simulink library "MCHP_Blockset"  (R2014b)
settings: Solver=ode45  SolverMode=SingleTasking  StartTime=0.0  StopTime=10.0  RelTol=1e-3
InitFcn:
  | disp('MCHP_Blockset_Library_InitFunction');
undefined symbols (not defined in the file): A0, A2, AD0, AVdd, B1, B5, B9, C10, C2, CMP2A, CMP3A, CMP4A, EXTREF1, EXTREF2, gcbh, MaxPer, MCHP_ACC_SAMx_Callback, MCHP_ADC_Callback, MCHP_ADC_HighSpeed_SAR_Callback, MCHP_ADC_HighSpeed_SAR_dsPIC_Callback, MCHP_ADC_SAME5x_Callback, MCHP_AFEC_SAM7x_Callback, MCHP_BUS_I2C_MASTER_callback, MCHP_BUS_SPI_callback, MCHP_C_function_Call_callback, MCHP_CN_Callback, MCHP_COMPARATOR1_callback, MCHP_CompilerOptimisation_Callback, MCHP_DACC_SAMx_Callback, MCHP_Digital_Input_Callback, MCHP_Digital_Output_Read_Callback, MCHP_Digital_Output_Write_Callback, MCHP_Fun, MCHP_HighSpeed_AnalogComparator_Callback, MCHP_IC_Callback, MCHP_IdleTask_Callback, MCHP_Interrupt_Callback, MCHP_Master_Callback, MCHP_MCPWM_Callback, MCHP_MCU_LOAD_Callback, MCHP_MCU_OVERLOAD_Callback, MCHP_MSI_Callback, MCHP_OC_HW_Callback, MCHP_OC_SW_Callback, MCHP_OP_AMP_Callback, MCHP_OrderInOut, MCHP_PDEC_Callback, MCHP_PGA_Callback, MCHP_PWM_Callback, MCHP_PWM_HighSpeed_Override_Callback, MCHP_PWM_HS_FEP_Callback, MCHP_PWM_SAM7x_Callback, MCHP_PWM_SAM7x_Override_Callback, MCHP_QDEC_SAMx_Callback, MCHP_QEI_Callback, MCHP_Scheduler_Options_Callback, MCHP_SECONDARY_CORE_Callback, MCHP_Tasks_State_Callback, MCHP_TCC_PWM_Callback, MCHP_TIMER_Config_Callback ... (+18)
libraries: MCHP_Blockset x2
(part 7 of 9)

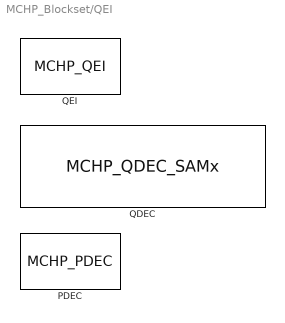
== system MCHP_Blockset/QEI ==
  PDEC : S-Function  InitFcn=MCHP_PDEC_Callback(gcb,'InitFcn');  FunctionName=MCHP_PDEC  Parameters=MCHP_PDEC_Callback(gcbh,'S_INPUT'),MCHP_PDEC_Callback(gcbh,'S_OUTPUT'),MCHP_PDEC_Callback(gcbh,'S_INPUT_Size'),MCHP_PDEC_Callback(gcbh,'S_OUTPUT_Size'),MCHP_PDEC_Callback(gcbh,'S_ListCustomDatatype'),SampleTime,0  EnableBusSupport=off  mask(PDEC){Mode=Quadrature Encoder, index=Reset counter, QDI0=PC16 / Pin[70], QDI0_txt=Dynamic Options, QDI1=PC17 / Pin[71], QDI1_txt=Dynamic Options, QDI2=PC18 / Pin[72], QDI2_txt=Dynamic Options, maxCounterReset=500, AutoCorrection=on, AutoCorrection_override=on, info=0, MCHP_MASTERLINK=SAME5x_PDEC_QEI_R2014b/Microchip Master, SampleTime=.01, MCHP_PORT={PDEC A}{QDI0}5:0:P80;{PDEC B}{QDI1}5:0:P81;{PDEC index}{QDI2}5:0:P82;, MAXPOS_INPUT=off, RESET_INPUT=off, OutputCounter=on, OutputCounter_Signed=unsigned, OutputRevolution=off, CounterRevolution_length=Counter is 13 bits ; revolution is 3 bits, OutputRevolution_Signed=unsigned, FILTER=2.55 (us)  ->  freq 196 (KHz), FILTER_TXT=2.55 (us)  ->  freq 196 (KHz), SWAP=off, QDI_invert_0=off, QDI_invert_1=off, QDI_invert_2=off}
      mask prompts: QDI0 "Phase A (QDI0)"; QDI0_txt "Signal 0"; QDI1 "Phase B (QDO1)"; QDI1_txt "Signal 1"; QDI2 "Index (QDI2)"; QDI2_txt "Signal 2"; maxCounterReset "Reset counter at value (-1 for never)"; AutoCorrection "Enable Auto-correction"; AutoCorrection_override "Enable Auto-correction"; SampleTime "Sample Time"; MAXPOS_INPUT "Max Counter is a block input"; RESET_INPUT "Reset Position and Counter on block input level"; OutputCounter "Output counter value"; OutputCounter_Signed "Output counter is"; OutputRevolution "Output revolution"; CounterRevolution_length "Length"; OutputRevolution_Signed "Output revolution is"; FILTER "Filter: min signal duration"; FILTER_TXT "Filter inputs"; SWAP "Swap pin phase A && B"; QDI_invert_0 "Invert Phase A logic (QDI0)"; QDI_invert_1 "Invert Phase B logic (QDI1)"; QDI_invert_2 "Invert index logic (QDI2)"
      mask help:
      | PDEC peripheral for SAM D5x / E5x / PIC32C
      |
      | Quadrature Encoder
      mask init:
      | MCHP_PDEC_Callback(gcbh,'INITIALISATION');
      settings: CopyFcn=MCHP_Fun.BlockUpdate(gcbh);  DeleteFcn=MCHP_PDEC_Callback(gcbh,'DeleteFcn');  OpenFcn=MCHP_PDEC_Callback(gcb,'OPEN');
      mask TypeOptions Mode: Quadrature Encoder | Counter with direction
      mask Callback Mode: MCHP_PDEC_Callback(gcbh,'UpdateGUI');
      mask TypeOptions index: Not used | Reset counter
      mask Callback index: MCHP_PDEC_Callback(gcbh,'UpdateGUI');
      mask TypeOptions QDI0: PA24 / Pin[94] | PB18 / Pin[84] | PB23 / Pin[99] | PC16 / Pin[70]
      mask TypeOptions QDI0_txt: Dynamic Options
      mask TypeOptions QDI1: PA25 / Pin[95] | PB19 / Pin[85] | PB24 / Pin[100] | PC17 / Pin[71]
      mask TypeOptions QDI1_txt: Dynamic Options
      mask TypeOptions QDI2: PB20 / Pin[86] | PB22 / Pin[98] | PB25 / Pin[101] | PC18 / Pin[72]
      mask TypeOptions QDI2_txt: Dynamic Options
      mask Callback MAXPOS_INPUT: MCHP_PDEC_Callback(gcbh,'UpdateGUI');
      mask TypeOptions OutputCounter_Signed: unsigned | signed
      mask Callback OutputRevolution: MCHP_PDEC_Callback(gcbh,'UpdateGUI');
      mask TypeOptions CounterRevolution_length: Counter is 16 bits ; no revolution | Counter is 15 bits ; revolution is 1 bit | Counter is 14 bits ; revolution is 2 bits | Counter is 13 bits ; revolution is 3 bits | Counter is 12 bits ; revolution is 4 bits | Counter is 11 bits ; revolution is 5 bits | Counter is 10 bits ; revolution is 6 bits | Counter is   9 bits ; revolution is 7 bits
      mask Callback CounterRevolution_length: MCHP_PDEC_Callback(gcbh,'UpdateGUI');
      mask TypeOptions OutputRevolution_Signed: unsigned | signed
      mask TypeOptions FILTER: disabled | 10 (ns)  ->  freq 50 (MHz) | 20 (ns)  ->  freq 25 (MHz) | 30 (ns)  ->  freq 16.7 (MHz) | 40 (ns)  ->  freq 12.5 (MHz) | 50 (ns)  ->  freq 10 (MHz) | 60 (ns)  ->  freq 8.33 (MHz) | 70 (ns)  ->  freq 7.14 (MHz) | 80 (ns)  ->  freq 6.25 (MHz) | 90 (ns)  ->  freq 5.56 (MHz) | 100 (ns)  ->  freq 5 (MHz) | 110 (ns)  ->  freq 4.55 (MHz) | 120 (ns)  ->  freq 4.17 (MHz) | 130 (ns)  ->  freq 3.85 (MHz) | 140 (ns)  ->  freq 3.57 (MHz) | 150 (ns)  ->  freq 3.33 (MHz) | 160 (ns)  ->  freq 3.13 (MHz) | 170 (ns)  ->  freq 2.94 (MHz) | 180 (ns)  ->  freq 2.78 (MHz) | 190 (ns)  ->  freq 2.63 (MHz) | 200 (ns)  ->  freq 2.5 (MHz) | 210 (ns)  ->  freq 2.38 (MHz) | 220 (ns)  ->  freq 2.27 (MHz) | 230 (ns)  ->  freq 2.17 (MHz) | 240 (ns)  ->  freq 2.08 (MHz) | 250 (ns)  ->  freq 2 (MHz) | 260 (ns)  ->  freq 1.92 (MHz) | 270 (ns)  ->  freq 1.85 (MHz) | 280 (ns)  ->  freq 1.79 (MHz) | 290 (ns)  ->  freq 1.72 (MHz) | 300 (ns)  ->  freq 1.67 (MHz) | 310 (ns)  ->  freq 1.61 (MHz) | 320 (ns)  ->  freq 1.56 (MHz) | 330 (ns)  ->  freq 1.52 (MHz) | 340 (ns)  ->  freq 1.47 (MHz) | 350 (ns)  ->  freq 1.43 (MHz) | 360 (ns)  ->  freq 1.39 (MHz) | 370 (ns)  ->  freq 1.35 (MHz) | 380 (ns)  ->  freq 1.32 (MHz) | 390 (ns)  ->  freq 1.28 (MHz) | 400 (ns)  ->  freq 1.25 (MHz) | 410 (ns)  ->  freq 1.22 (MHz) | 420 (ns)  ->  freq 1.19 (MHz) | 430 (ns)  ->  freq 1.16 (MHz) | 440 (ns)  ->  freq 1.14 (MHz) | 450 (ns)  ->  freq 1.11 (MHz) | 460 (ns)  ->  freq 1.09 (MHz) | 470 (ns)  ->  freq 1.06 (MHz) | 480 (ns)  ->  freq 1.04 (MHz) | 490 (ns)  ->  freq 1.02 (MHz) | 500 (ns)  ->  freq 1e+03 (KHz) | 510 (ns)  ->  freq 980 (KHz) | 520 (ns)  ->  freq 962 (KHz) | 530 (ns)  ->  freq 943 (KHz) | 540 (ns)  ->  freq 926 (KHz) | 550 (ns)  ->  freq 909 (KHz) | 560 (ns)  ->  freq 893 (KHz) | 570 (ns)  ->  freq 877 (KHz) | 580 (ns)  ->  freq 862 (KHz) | 590 (ns)  ->  freq 847 (KHz) | 600 (ns)  ->  freq 833 (KHz) | 610 (ns)  ->  freq 820 (KHz) | 620 (ns)  ->  freq 806 (KHz) | 630 (ns)  ->  freq 794 (KHz) | 640 (ns)  ->  freq 781 (KHz) | 650 (ns)  ->  freq 769 (KHz) | 660 (ns)  ->  freq 758 (KHz) | 670 (ns)  ->  freq 746 (KHz) | 680 (ns)  ->  freq 735 (KHz) | 690 (ns)  ->  freq 725 (KHz) | 700 (ns)  ->  freq 714 (KHz) | 710 (ns)  ->  freq 704 (KHz) | 720 (ns)  ->  freq 694 (KHz) | 730 (ns)  ->  freq 685 (KHz) | 740 (ns)  ->  freq 676 (KHz) | 750 (ns)  ->  freq 667 (KHz) | 760 (ns)  ->  freq 658 (KHz) | 770 (ns)  ->  freq 649 (KHz) | 780 (ns)  ->  freq 641 (KHz) | 790 (ns)  ->  freq 633 (KHz) | 800 (ns)  ->  freq 625 (KHz) | 810 (ns)  ->  freq 617 (KHz) | 820 (ns)  ->  freq 610 (KHz) | 830 (ns)  ->  freq 602 (KHz) | 840 (ns)  ->  freq 595 (KHz) | 850 (ns)  ->  freq 588 (KHz) | 860 (ns)  ->  freq 581 (KHz) | 870 (ns)  ->  freq 575 (KHz) | 880 (ns)  ->  freq 568 (KHz) | 890 (ns)  ->  freq 562 (KHz) | 900 (ns)  ->  freq 556 (KHz) | 910 (ns)  ->  freq 549 (KHz) | 920 (ns)  ->  freq 543 (KHz) | 930 (ns)  ->  freq 538 (KHz) | 940 (ns)  ->  freq 532 (KHz) | 950 (ns)  ->  freq 526 (KHz) | 960 (ns)  ->  freq 521 (KHz) | 970 (ns)  ->  freq 515 (KHz) | 980 (ns)  ->  freq 510 (KHz) | 990 (ns)  ->  freq 505 (KHz) | 1e+03 (ns)  ->  freq 500 (KHz) | 1.01 (us)  ->  freq 495 (KHz) | 1.02 (us)  ->  freq 490 (KHz) | 1.03 (us)  ->  freq 485 (KHz) | 1.04 (us)  ->  freq 481 (KHz) | 1.05 (us)  ->  freq 476 (KHz) | 1.06 (us)  ->  freq 472 (KHz) | 1.07 (us)  ->  freq 467 (KHz) | 1.08 (us)  ->  freq 463 (KHz) | 1.09 (us)  ->  freq 459 (KHz) | 1.1 (us)  ->  freq 455 (KHz) | 1.11 (us)  ->  freq 450 (KHz) | 1.12 (us)  ->  freq 446 (KHz) | 1.13 (us)  ->  freq 442 (KHz) | 1.14 (us)  ->  freq 439 (KHz) | 1.15 (us)  ->  freq 435 (KHz) | 1.16 (us)  ->  freq 431 (KHz) | 1.17 (us)  ->  freq 427 (KHz) | 1.18 (us)  ->  freq 424 (KHz) | 1.19 (us)  ->  freq 420 (KHz) | 1.2 (us)  ->  freq 417 (KHz) | 1.21 (us)  ->  freq 413 (KHz) | 1.22 (us)  ->  freq 410 (KHz) | 1.23 (us)  ->  freq 407 (KHz) | 1.24 (us)  ->  freq 403 (KHz) | 1.25 (us)  ->  freq 400 (KHz) | 1.26 (us)  ->  freq 397 (KHz) | 1.27 (us)  ->  freq 394 (KHz) | 1.28 (us)  ->  freq 391 (KHz) | 1.29 (us)  ->  freq 388 (KHz) | 1.3 (us)  ->  freq 385 (KHz) | 1.31 (us)  ->  freq 382 (KHz) | 1.32 (us)  ->  freq 379 (KHz) | 1.33 (us)  ->  freq 376 (KHz) | 1.34 (us)  ->  freq 373 (KHz) | 1.35 (us)  ->  freq 370 (KHz) | 1.36 (us)  ->  freq 368 (KHz) | 1.37 (us)  ->  freq 365 (KHz) | 1.38 (us)  ->  freq 362 (KHz) | 1.39 (us)  ->  freq 360 (KHz) | 1.4 (us)  ->  freq 357 (KHz) | 1.41 (us)  ->  freq 355 (KHz) | 1.42 (us)  ->  freq 352 (KHz) | 1.43 (us)  ->  freq 350 (KHz) | 1.44 (us)  ->  freq 347 (KHz) | 1.45 (us)  ->  freq 345 (KHz) | 1.46 (us)  ->  freq 342 (KHz) | 1.47 (us)  ->  freq 340 (KHz) | 1.48 (us)  ->  freq 338 (KHz) | 1.49 (us)  ->  freq 336 (KHz) | 1.5 (us)  ->  freq 333 (KHz) | 1.51 (us)  ->  freq 331 (KHz) | 1.52 (us)  ->  freq 329 (KHz) | 1.53 (us)  ->  freq 327 (KHz) | 1.54 (us)  ->  freq 325 (KHz) | 1.55 (us)  ->  freq 323 (KHz) | 1.56 (us)  ->  freq 321 (KHz) | 1.57 (us)  ->  freq 318 (KHz) | 1.58 (us)  ->  freq 316 (KHz) | 1.59 (us)  ->  freq 314 (KHz) | 1.6 (us)  ->  freq 313 (KHz) | 1.61 (us)  ->  freq 311 (KHz) | 1.62 (us)  ->  freq 309 (KHz) | 1.63 (us)  ->  freq 307 (KHz) | 1.64 (us)  ->  freq 305 (KHz) | 1.65 (us)  ->  freq 303 (KHz) | 1.66 (us)  ->  freq 301 (KHz) | 1.67 (us)  ->  freq 299 (KHz) | 1.68 (us)  ->  freq 298 (KHz) | 1.69 (us)  ->  freq 296 (KHz) | 1.7 (us)  ->  freq 294 (KHz) | 1.71 (us)  ->  freq 292 (KHz) | 1.72 (us)  ->  freq 291 (KHz) | 1.73 (us)  ->  freq 289 (KHz) | 1.74 (us)  ->  freq 287 (KHz) | 1.75 (us)  ->  freq 286 (KHz) | 1.76 (us)  ->  freq 284 (KHz) | 1.77 (us)  ->  freq 282 (KHz) | 1.78 (us)  ->  freq 281 (KHz) | 1.79 (us)  ->  freq 279 (KHz) | 1.8 (us)  ->  freq 278 (KHz) | 1.81 (us)  ->  freq 276 (KHz) | 1.82 (us)  ->  freq 275 (KHz) | 1.83 (us)  ->  freq 273 (KHz) | 1.84 (us)  ->  freq 272 (KHz) | 1.85 (us)  ->  freq 270 (KHz) | 1.86 (us)  ->  freq 269 (KHz) | 1.87 (us)  ->  freq 267 (KHz) | 1.88 (us)  ->  freq 266 (KHz) | 1.89 (us)  ->  freq 265 (KHz) | 1.9 (us)  ->  freq 263 (KHz) | 1.91 (us)  ->  freq 262 (KHz) | 1.92 (us)  ->  freq 260 (KHz) | 1.93 (us)  ->  freq 259 (KHz) | 1.94 (us)  ->  freq 258 (KHz) | 1.95 (us)  ->  freq 256 (KHz) | 1.96 (us)  ->  freq 255 (KHz) | 1.97 (us)  ->  freq 254 (KHz) | 1.98 (us)  ->  freq 253 (KHz) | 1.99 (us)  ->  freq 251 (KHz) | 2 (us)  ->  freq 250 (KHz) | 2.01 (us)  ->  freq 249 (KHz) | 2.02 (us)  ->  freq 248 (KHz) | 2.03 (us)  ->  freq 246 (KHz) | 2.04 (us)  ->  freq 245 (KHz) | 2.05 (us)  ->  freq 244 (KHz) | 2.06 (us)  ->  freq 243 (KHz) | 2.07 (us)  ->  freq 242 (KHz) | 2.08 (us)  ->  freq 240 (KHz) | 2.09 (us)  ->  freq 239 (KHz) | 2.1 (us)  ->  freq 238 (KHz) | 2.11 (us)  ->  freq 237 (KHz) | 2.12 (us)  ->  freq 236 (KHz) | 2.13 (us)  ->  freq 235 (KHz) | 2.14 (us)  ->  freq 234 (KHz) | 2.15 (us)  ->  freq 233 (KHz) | 2.16 (us)  ->  freq 231 (KHz) | 2.17 (us)  ->  freq 230 (KHz) | 2.18 (us)  ->  freq 229 (KHz) | 2.19 (us)  ->  freq 228 (KHz) | 2.2 (us)  ->  freq 227 (KHz) | 2.21 (us)  ->  freq 226 (KHz) | 2.22 (us)  ->  freq 225 (KHz) | 2.23 (us)  ->  freq 224 (KHz) | 2.24 (us)  ->  freq 223 (KHz) | 2.25 (us)  ->  freq 222 (KHz) | 2.26 (us)  ->  freq 221 (KHz) | 2.27 (us)  ->  freq 220 (KHz) | 2.28 (us)  ->  freq 219 (KHz) | 2.29 (us)  ->  freq 218 (KHz) | 2.3 (us)  ->  freq 217 (KHz) | 2.31 (us)  ->  freq 216 (KHz) | 2.32 (us)  ->  freq 216 (KHz) | 2.33 (us)  ->  freq 215 (KHz) | 2.34 (us)  ->  freq 214 (KHz) | 2.35 (us)  ->  freq 213 (KHz) | 2.36 (us)  ->  freq 212 (KHz) | 2.37 (us)  ->  freq 211 (KHz) | 2.38 (us)  ->  freq 210 (KHz) | 2.39 (us)  ->  freq 209 (KHz) | 2.4 (us)  ->  freq 208 (KHz) | 2.41 (us)  ->  freq 207 (KHz) | 2.42 (us)  ->  freq 207 (KHz) | 2.43 (us)  ->  freq 206 (KHz) | 2.44 (us)  ->  freq 205 (KHz) | 2.45 (us)  ->  freq 204 (KHz) | 2.46 (us)  ->  freq 203 (KHz) | 2.47 (us)  ->  freq 202 (KHz) | 2.48 (us)  ->  freq 202 (KHz) | 2.49 (us)  ->  freq 201 (KHz) | 2.5 (us)  ->  freq 200 (KHz) | 2.51 (us)  ->  freq 199 (KHz) | 2.52 (us)  ->  freq 198 (KHz) | 2.53 (us)  ->  freq 198 (KHz) | 2.54 (us)  ->  freq 197 (KHz) | 2.55 (us)  ->  freq 196 (KHz)
      mask Display:
      | MCHP_DrawLogo;fprintf('PDEC');
      | port_label('output', 1 ,' count ');
  QDEC : S-Function  InitFcn=MCHP_QDEC_SAMx_Callback(gcbh,'InitFcn');  FunctionName=MCHP_QDEC_SAMx  Parameters=MCHP_QDEC_SAMx_Callback(gcbh,'S_INPUT'),MCHP_QDEC_SAMx_Callback(gcbh,'S_OUTPUT'),MCHP_QDEC_SAMx_Callback(gcbh,'S_INPUT_Size'),MCHP_QDEC_SAMx_Callback(gcbh,'S_OUTPUT_Size'),MCHP_QDEC_SAMx_Callback(gcbh,'S_INPUT_FeedThrough'),0,SampleTime,0  EnableBusSupport=off  mask(Ouput Driver for Quadrature Decoder (QDEC)){QDEC_REF=Dynamic Options, QDEC_REF_TXT=TC0, PHA_PIN=Dynamic Options, PHA_PIN_TXT=PA0 / Pin[102], PHB_PIN=Dynamic Options, PHB_PIN_TXT=PA1 / Pin[99], IDX_PIN=Dynamic Options, IDX_PIN_TXT=PA16 / Pin[45], INVERT_PHA=off, INVERT_PHB=off, INVERT_IDX=on, SWAP_PHA_PHB=off, SampleTime=.001, MCHP_PORT={TC0}{TIOA0}3:0:P0;{TC0}{TIOB0}3:0:P1;{TC0}{TIOB1}3:0:P16;, MCHP_MASTERLINK=SAMx7_MCLV2_QDEC_Testing_R2014b/Microchip Master, MCHP_TIMER_REQUEST={Quadrature Decoder (Phase Counter)}{QDEC0}20:4:4:0:[1]:65535;{Quadrature Decoder (IDX Counter)}{QDEC0}20:4:4:0:[2]:65535;{Quadrature Decoder (Speed Measurement Time Base)}{QDEC0}20:4:4:0:[3]:65535;, MCHP_TIMER_RESULT=[0 -0.5 ;2 65533.999999999985448 ;3 65533.999999999985448 ], QDEC_MODE=Position, POSITION_OUTPUT=is a 16 bits signed block output, INDEX_OUTPUT=is not a block output, RESET_INPUT=off, POSITION_RESET_MODE=on each IDX signal, RESET_EDGE=rising edge, POSITION_RESET_VALUE=1000, SPEED_TIME_BASE=Dynamic Options, SPEED_TIME_BASE_TXT=Resol: 666.7(ns) - MaxPer: 43.7(ms), SPEED_OUTPUT=is a 16 bits unsigned block output, DIR_OUTPUT=is a boolean block output, DIRCHG_OUTPUT=is a boolean block output, AUTO_CORRECTION=on, MAX_PERIOD_FILTER=Dynamic Options, MAX_PERIOD_FILTER_TXT=4(us), MAXCMP=disabled, MPE_OUTPUT=is not a block output, QERR_OUTPUT=is not a block output}
      mask prompts: QDEC_REF "QDEC set on Timer Counter"; QDEC_REF_TXT "QDEC_REF"; PHA_PIN "Phase A Input Signal (PHA)"; PHB_PIN "Phase B Input Signal (PHB)"; IDX_PIN "Index Input Signal (IDX)"; INVERT_PHA "Invert PHA"; INVERT_PHB "Invert PHB"; INVERT_IDX "Invert IDX"; SWAP_PHA_PHB "Swap PHA and PHB"; SampleTime "Sample Time"; QDEC_MODE "QDEC Mode"; POSITION_OUTPUT "Pulse Counter (Absolute Position)"; INDEX_OUTPUT "Index Counter (Number of rotations)"; RESET_INPUT "Reset Position and Index Counters on block input level"; POSITION_RESET_MODE "Position Reset Mode"; RESET_EDGE "Reset Position on IDX signal"; POSITION_RESET_VALUE "Position Reset Value  (range [0  65535])"; SPEED_TIME_BASE "Speed Measurement time base"; SPEED_TIME_BASE_TXT "SPEED_TIME_BASE"; SPEED_OUTPUT "Speed"; DIR_OUTPUT "Direction Status"; DIRCHG_OUTPUT "Rotation Change Detection Flag"; AUTO_CORRECTION "Enable AutoCorrection of missing pulses"; MAX_PERIOD_FILTER "Filter phase pulses with a period shorter than"; MAXCMP "Maximum Consecutive Missing Pulses allowed"; MPE_OUTPUT "Consecutive Missing Pulse Error Flag"; QERR_OUTPUT "Quadrature Error Flag"
      mask help:
      | The Quadrature Decoder (QDEC) is connected in front of the Timer-Counter module (TC). When enabled, the QDEC performs the input lines filtering, decoding of quadrature signals and connects to the Timers-Counters in order to read the position or speed of the motor.
      |
      | Either speed or position/revolution can be measured. If enabled, the Pulse Counter for Index signal (IDX) can be read in any mode.
      mask init:
      | MCHP_QDEC_SAMx_Callback(gcbh,'INITIALISATION');
      settings: PreSaveFcn=MCHP_Fun.PreSaveFcn_DynamicOptions(gcbh);  OpenFcn=MCHP_QDEC_SAMx_Callback(gcbh,'OPEN');
      mask TypeOptions QDEC_REF: Dynamic Options
      mask Callback QDEC_REF: MCHP_QDEC_SAMx_Callback(gcbh,'INITIALISATION');
      mask TypeOptions PHA_PIN: Dynamic Options
      mask TypeOptions PHB_PIN: Dynamic Options
      mask TypeOptions IDX_PIN: Dynamic Options
      mask TypeOptions QDEC_MODE: Position | Speed
      mask Callback QDEC_MODE: MCHP_QDEC_SAMx_Callback(gcbh,'UpdateGUI');
      mask TypeOptions POSITION_OUTPUT: is a 16 bits unsigned block output | is a 16 bits signed block output | is a 32 bits unsigned block output | is a 32 bits signed block output
      mask TypeOptions INDEX_OUTPUT: is not a block output | is a 16 bits unsigned block output | is a 16 bits signed block output | is a 32 bits unsigned block output | is a 32 bits signed block output
      mask Callback INDEX_OUTPUT: MCHP_QDEC_SAMx_Callback(gcbh,'UpdateGUI');
      mask TypeOptions POSITION_RESET_MODE: never reset position | on each IDX signal | at user defined value
      mask Callback POSITION_RESET_MODE: MCHP_QDEC_SAMx_Callback(gcbh,'UpdateGUI');
      mask TypeOptions RESET_EDGE: rising edge | falling edge | depends on a RST_EDGE block input :1 rising / 0 falling
      mask TypeOptions SPEED_TIME_BASE: Dynamic Options
      mask TypeOptions SPEED_OUTPUT: is a 16 bits unsigned block output | is a 32 bits unsigned block output
      mask TypeOptions DIR_OUTPUT: is not a block output | is a boolean block output
      mask TypeOptions DIRCHG_OUTPUT: is not a block output | is a boolean block output
      mask TypeOptions MAX_PERIOD_FILTER: Dynamic Options
      mask TypeOptions MAXCMP: disabled | 1 | 2 | 3 | 4 | 5 | 6 | 7 | 8 | 9 | 10 | 11 | 12 | 13 | 14 | 15
      mask TypeOptions MPE_OUTPUT: is not a block output | is a boolean block output
      mask TypeOptions QERR_OUTPUT: is not a block output | is a boolean block output
      mask Display:
      | fprintf('QDEC (TC%u)', 0);
      | port_label('output',1,'Pulse Counter');
      | port_label('output',2,'Direction Status');
      | port_label('output',3,'Rotation Change Flag');
  QEI : S-Function  LoadFcn=MCHP_Fun.Load_EvalIn_ws(gcbh);  InitFcn=MCHP_QEI_Callback(gcbh,'InitFcn');  FunctionName=MCHP_QEI  Parameters=SampleTime,MCHP_QEI_Callback(gcbh,'S_INPUT'),MCHP_QEI_Callback(gcbh,'S_OUTPUT'),0  EnableBusSupport=off  mask(Output Driver for Quadrature Encoder Interface (QEI) peripheral){QEI_REF=1, QEI_MODE=Quadrature Encoder, QEI_x2mode=off, QEI_PulseCountDir=Down, PIN_QEA=Dynamic Options, PIN_QEA_TXT=Dynamic Options, PIN_QEB=Dynamic Options, PIN_QEB_TXT=Dynamic Options, SWPAB=off, QEAPOL=off, QEBPOL=off, SampleTime=.001, PIN_CCMP=Dynamic Options, PIN_CCMP_TXT=Dynamic Options, evalin_ws='', MCHP_PORT={QEI1 A}{QEA1}5:0:B4;{QEI1 B}{QEB1}5:0:B5;, MCHP_MASTERLINK=QEI_30f3010_PICDEM_MCLV/Microchip Master, INDXxCNT_Output=is not an output, POSxCNT_Output=is a 16 bits unsigned block output, RESET_Input=off, PIMOD_mode=Never reset position, PIMOD_modeB=Never reset position, PIMOD_reset=on next INDEX event, PIN_INDEX=Dynamic Options, PIN_INDEX_TXT=Dynamic Options, IMV=QEA = 1 and QEB = 0, IMV_x2=QEA = 1, PIN_HOME=Dynamic Options, PIN_HOME_TXT=Dynamic Options, QEIxLEC_GEC=[0 200], QEIxIC=52, PCIIRQ=off, IDXPOL=off, HOMPOL=on, VELxCNT_Output=is a 16 bits unsigned block output, INTxHLD_Output=is not an output, MaxPeriod=1e-3, FILTREN=on, QFDIV_popup=Dynamic Options, QFDIV_popup_TXT=26.04 kHz, FILTER_CutOffFreq=100e3, QEI_IntPri=5}
      mask prompts: QEI_REF "QEI"; QEI_MODE "Mode"; QEI_x2mode "Divide resolution by a factor 2"; QEI_PulseCountDir "Counting Direction"; PIN_QEA "QEA Input Signal"; PIN_QEA_TXT "pin QEA"; PIN_QEB "QEB Input Signal"; PIN_QEB_TXT "pin QEB"; SWPAB "Reverse Direction (SWAP QEA and QEB)"; QEAPOL "Invert QEA Polarity"; QEBPOL "Invert QEB Polarity"; SampleTime "Sample Time"; PIN_CCMP "Comparator output signal"; PIN_CCMP_TXT "pin Output"; INDXxCNT_Output "Index counter (Number of completed rotation)"; POSxCNT_Output "Position (Absolute)"; RESET_Input "Reset block input Re-Initialise Position (on input level)"; PIMOD_mode "Position : reset / modulo"; PIMOD_modeB "Position : reset / modulo"; PIMOD_reset "user define reset event:"; PIN_INDEX "INDEX Input Signal"; PIN_INDEX_TXT "pin INDEX"; IMV "Index event is asserted when INDEX signal = 1 AND"; IMV_x2 "Index event is asserted when INDEX signal = 1 AND"; PIN_HOME "HOME Input Signal"; PIN_HOME_TXT "pin HOME"; QEIxLEC_GEC "modulo : [ 0   High ] reset when reaching High value    (range [+0   +65535])"; QEIxIC "Position Initialisation Value: (range [+0   +65535])"; PCIIRQ "Initialisation Status is a block Output"; IDXPOL "Invert INDEX Polarity"; HOMPOL "Invert HOME Polarity"; VELxCNT_Output "Velocity Counter :  Position * ( 1-1/z )"; INTxHLD_Output "Period between each count pulses"; MaxPeriod "Max period between count pulse (Resolution: 4.8e-08s  ;  QEI1max=  2^14.36 )"; FILTREN "Filter Inputs Signals (Activate Triple Sampling)"; QFDIV_popup "Filter cut off freq (set above 1/2 of the max POSCNT rate)"; FILTER_CutOffFreq "Filter Cut off freq (Hz)  ==> Closest value found:  156250Hz"; QEI_IntPri "QEI Interruption Priority"
      mask help: Measure position and/or speed
      mask init:
      | MCHP_QEI_Callback(gcbh,'INITIALISATION');
      settings: PreSaveFcn=MCHP_Fun.PreSaveFcn_DynamicOptions(gcbh);  OpenFcn=MCHP_QEI_Callback(gcbh,'OPEN');
      mask TypeOptions QEI_REF: 1 | 2 | 3 | 4 | 5 | 6 | 7 | 8 | 9
      mask Callback QEI_REF: MCHP_QEI_Callback(gcbh,'QEI_REF');
      mask TypeOptions QEI_MODE: Quadrature Encoder | External Pulse Counter | External Pulse Counter with Direction (Up/Down) Input
      mask Callback QEI_MODE: MCHP_QEI_Callback(gcbh,'QEI_MODE');
      mask Callback QEI_x2mode: MCHP_QEI_Callback(gcbh,'QEI_x2mode');
      mask TypeOptions QEI_PulseCountDir: Up | Down
      mask TypeOptions PIN_QEA: Dynamic Options
      mask Callback PIN_QEA: MCHP_QEI_Callback(gcbh,'PIN_QEA');
      mask TypeOptions PIN_QEB: Dynamic Options
      mask Callback PIN_QEB: MCHP_QEI_Callback(gcbh,'PIN_QEB');
      mask Callback SWPAB: MCHP_QEI_Callback(gcbh,'SWPAB');
      mask TypeOptions PIN_CCMP: Dynamic Options
      mask Callback PIN_CCMP: MCHP_QEI_Callback(gcbh,'PIN_CCMP');
      mask TypeOptions INDXxCNT_Output: is not an output | is a 16 bits unsigned block output | is a 16 bits signed block output
      mask Callback INDXxCNT_Output: MCHP_QEI_Callback(gcbh,'INDXxCNT_Output');
      mask TypeOptions POSxCNT_Output: is not an output | is a 16 bits unsigned block output | is a 16 bits signed block output
      mask Callback POSxCNT_Output: MCHP_QEI_Callback(gcbh,'POSxCNT_Output');
      mask Callback RESET_Input: MCHP_QEI_Callback(gcbh,'RESET_Input');
      mask TypeOptions PIMOD_mode: Never reset position | position is cyclique between user defined boundaries | position is cyclique between user defined boundaries and RESET position on each INDEX event | RESET position on each INDEX event | RESET position when value reach a user defined boundarie | INITIALISE position value once on user define reset event
      mask Callback PIMOD_mode: MCHP_QEI_Callback(gcbh,'PIMOD_mode');
      mask TypeOptions PIMOD_modeB: Never reset position | RESET position on each INDEX event | RESET position when value reach a user defined boundarie
      mask Callback PIMOD_modeB: MCHP_QEI_Callback(gcbh,'PIMOD_modeB');
      mask TypeOptions PIMOD_reset: on next INDEX event | on next on next INDEX event following a HOME input | on second detect of INDEX event following a HOME input
      mask Callback PIMOD_reset: MCHP_QEI_Callback(gcbh,'PIMOD_reset');
      mask TypeOptions PIN_INDEX: Dynamic Options
      mask Callback PIN_INDEX: MCHP_QEI_Callback(gcbh,'PIN_INDEX');
      mask TypeOptions IMV: QEA = 1 and QEB = 1 | QEA = 0 and QEB = 1 | QEA = 1 and QEB = 0 | QEA = 0 and QEB = 0
      mask TypeOptions IMV_x2: QEA = 1 | QEA = 0 | QEB = 1 | QEB = 0
      mask TypeOptions PIN_HOME: Dynamic Options
      mask Callback PIN_HOME: MCHP_QEI_Callback(gcbh,'PIN_HOME');
      mask TypeOptions VELxCNT_Output: is not an output | is a 16 bits unsigned block output | is a 16 bits signed block output
      mask TypeOptions INTxHLD_Output: is not an output | is a 16 bits unsigned block output | is a 32 bits unsigned block output
      mask Callback FILTREN: MCHP_QEI_Callback(gcbh,'FILTREN');
      mask TypeOptions QFDIV_popup: Dynamic Options
      mask Callback QFDIV_popup: MCHP_QEI_Callback(gcbh,'QFDIV_popup');
      mask TypeOptions QEI_IntPri: 1 | 2 | 3 | 4 | 5 | 6 | 7
      mask Display:
      | MCHP_DrawLogo;
      | fprintf('QEI 1');
      | port_label('output',1,'POS');
